simulink model "test"  (R2016b)
settings: Solver=ode3  StartTime=0.0  StopTime=inf  FixedStep=0.01  RelTol=1e-3  EnableMultiTasking=on
undefined symbols (not defined in the file): C, D, eps_c, k_cc, K_q1f, K_q1r, K_q2f, K_q2r, K_q3f, K_q3r, K_q4f, K_q4r, K_q5f, K_q5r, K_q6f, K_q6r, K_T1f, K_T1r, K_T2f, K_T2r, K_T3f, K_T3r, K_T4f, K_T4r, K_T5f, K_T5r, K_T6f, K_T6r, Max_rotation, Max_thrust, Min_thrust, n_c, p_cc, pwm_thr1_backward, pwm_thr1_forward, pwm_thr2_backward, pwm_thr2_forward, pwm_thr3_backward, pwm_thr3_forward, pwm_thr4_backward, pwm_thr4_forward, pwm_thr5_backward, pwm_thr5_forward, pwm_thr6_backward, pwm_thr6_forward, r_cc, Rho, Thruster
libraries: dspmtrx3 x9, marine_gnc x8, simulink_extras x3, simulink x1
(part 3 of 4)

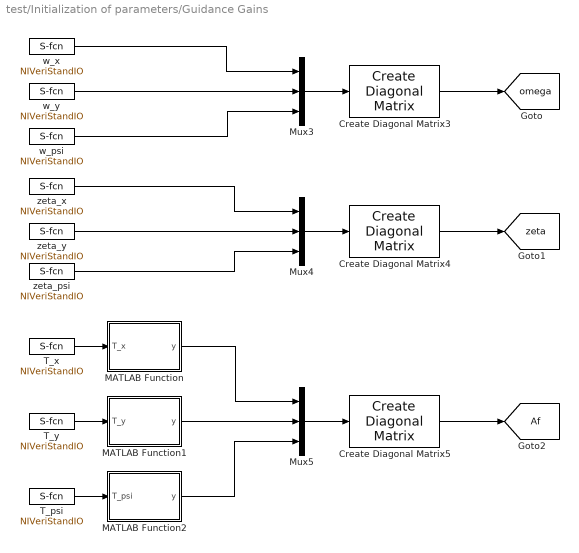
== system test/Initialization of parameters/Guidance Gains ==
  Create Diagonal Matrix3 : dspmtrx3/Create Diagonal Matrix
  Create Diagonal Matrix4 : dspmtrx3/Create Diagonal Matrix
  Create Diagonal Matrix5 : dspmtrx3/Create Diagonal Matrix
  MATLAB Function : MATLAB Function  TreatAsAtomicUnit=on
  MATLAB Function1 : MATLAB Function  TreatAsAtomicUnit=on
  MATLAB Function2 : MATLAB Function  TreatAsAtomicUnit=on
  Mux3 : Mux  Inputs=3
  Mux4 : Mux  Inputs=3
  Mux5 : Mux  Inputs=3
  T_psi : S-Function  Priority=7  FunctionName=NIVeriStandIO  Parameters=width dtype portnum stime stype btype  SFunctionDeploymentMode=off  EnableBusSupport=off  mask(NI VeriStand Inport){portnum=7, width=-1, stime=-1, dtype=auto, stype=auto, btype=1}
      mask prompts: portnum "Port number:"; width "Port dimensions (-1 for dynamically sized):"; stime "Sample time (-1 for inherited):"; dtype "Data type:"; stype "Signal type:"; btype "Block type:"
      mask help: Use this inport on any level of nested subsystems to allow NI VeriStand software to map signals to it.
      mask init:
      | NIVeriStandIO_init;
      settings: CopyFcn=NIVeriStand_MDL_functions('', 'IO_copy');  DeleteFcn=NIVeriStand_MDL_functions('', 'IO_delete');  MoveFcn=set_param(gcb, 'Mask', 'on');
      mask Callback portnum: NIVeriStand_MDL_functions('', 'IO_setportnum');
      mask TypeOptions dtype: auto | double | single | int8 | uint8 | int16 | uint16 | int32 | uint32 | boolean
      mask Callback dtype: NIVeriStand_MDL_functions('', 'IO_booleansignal');
      mask TypeOptions stype: auto | real | complex
      mask Display:
      | patch([-x x], [-y y], [.90980 .81960 .32156]);
      | plot([xrad -x x xrad], [yrad -y y yrad]);
      | fprintf('NI In%d', portnum);
  T_x : S-Function  Priority=8  FunctionName=NIVeriStandIO  Parameters=width dtype portnum stime stype btype  SFunctionDeploymentMode=off  EnableBusSupport=off  mask(NI VeriStand Inport){portnum=8, width=-1, stime=-1, dtype=auto, stype=auto, btype=1}
      mask prompts: portnum "Port number:"; width "Port dimensions (-1 for dynamically sized):"; stime "Sample time (-1 for inherited):"; dtype "Data type:"; stype "Signal type:"; btype "Block type:"
      mask help: Use this inport on any level of nested subsystems to allow NI VeriStand software to map signals to it.
      mask init:
      | NIVeriStandIO_init;
      settings: CopyFcn=NIVeriStand_MDL_functions('', 'IO_copy');  DeleteFcn=NIVeriStand_MDL_functions('', 'IO_delete');  MoveFcn=set_param(gcb, 'Mask', 'on');
      mask Callback portnum: NIVeriStand_MDL_functions('', 'IO_setportnum');
      mask TypeOptions dtype: auto | double | single | int8 | uint8 | int16 | uint16 | int32 | uint32 | boolean
      mask Callback dtype: NIVeriStand_MDL_functions('', 'IO_booleansignal');
      mask TypeOptions stype: auto | real | complex
      mask Display:
      | patch([-x x], [-y y], [.90980 .81960 .32156]);
      | plot([xrad -x x xrad], [yrad -y y yrad]);
      | fprintf('NI In%d', portnum);
  T_y : S-Function  Priority=9  FunctionName=NIVeriStandIO  Parameters=width dtype portnum stime stype btype  SFunctionDeploymentMode=off  EnableBusSupport=off  mask(NI VeriStand Inport){portnum=9, width=-1, stime=-1, dtype=auto, stype=auto, btype=1}
      mask prompts: portnum "Port number:"; width "Port dimensions (-1 for dynamically sized):"; stime "Sample time (-1 for inherited):"; dtype "Data type:"; stype "Signal type:"; btype "Block type:"
      mask help: Use this inport on any level of nested subsystems to allow NI VeriStand software to map signals to it.
      mask init:
      | NIVeriStandIO_init;
      settings: CopyFcn=NIVeriStand_MDL_functions('', 'IO_copy');  DeleteFcn=NIVeriStand_MDL_functions('', 'IO_delete');  MoveFcn=set_param(gcb, 'Mask', 'on');
      mask Callback portnum: NIVeriStand_MDL_functions('', 'IO_setportnum');
      mask TypeOptions dtype: auto | double | single | int8 | uint8 | int16 | uint16 | int32 | uint32 | boolean
      mask Callback dtype: NIVeriStand_MDL_functions('', 'IO_booleansignal');
      mask TypeOptions stype: auto | real | complex
      mask Display:
      | patch([-x x], [-y y], [.90980 .81960 .32156]);
      | plot([xrad -x x xrad], [yrad -y y yrad]);
      | fprintf('NI In%d', portnum);
  w_psi : S-Function  Priority=3  FunctionName=NIVeriStandIO  Parameters=width dtype portnum stime stype btype  SFunctionDeploymentMode=off  EnableBusSupport=off  mask(NI VeriStand Inport){portnum=3, width=-1, stime=-1, dtype=auto, stype=auto, btype=1}
      mask prompts: portnum "Port number:"; width "Port dimensions (-1 for dynamically sized):"; stime "Sample time (-1 for inherited):"; dtype "Data type:"; stype "Signal type:"; btype "Block type:"
      mask help: Use this inport on any level of nested subsystems to allow NI VeriStand software to map signals to it.
      mask init:
      | NIVeriStandIO_init;
      settings: CopyFcn=NIVeriStand_MDL_functions('', 'IO_copy');  DeleteFcn=NIVeriStand_MDL_functions('', 'IO_delete');  MoveFcn=set_param(gcb, 'Mask', 'on');
      mask Callback portnum: NIVeriStand_MDL_functions('', 'IO_setportnum');
      mask TypeOptions dtype: auto | double | single | int8 | uint8 | int16 | uint16 | int32 | uint32 | boolean
      mask Callback dtype: NIVeriStand_MDL_functions('', 'IO_booleansignal');
      mask TypeOptions stype: auto | real | complex
      mask Display:
      | patch([-x x], [-y y], [.90980 .81960 .32156]);
      | plot([xrad -x x xrad], [yrad -y y yrad]);
      | fprintf('NI In%d', portnum);
  w_x : S-Function  Priority=1  FunctionName=NIVeriStandIO  Parameters=width dtype portnum stime stype btype  SFunctionDeploymentMode=off  EnableBusSupport=off  mask(NI VeriStand Inport){portnum=1, width=-1, stime=-1, dtype=auto, stype=auto, btype=1}
      mask prompts: portnum "Port number:"; width "Port dimensions (-1 for dynamically sized):"; stime "Sample time (-1 for inherited):"; dtype "Data type:"; stype "Signal type:"; btype "Block type:"
      mask help: Use this inport on any level of nested subsystems to allow NI VeriStand software to map signals to it.
      mask init:
      | NIVeriStandIO_init;
      settings: CopyFcn=NIVeriStand_MDL_functions('', 'IO_copy');  DeleteFcn=NIVeriStand_MDL_functions('', 'IO_delete');  MoveFcn=set_param(gcb, 'Mask', 'on');
      mask Callback portnum: NIVeriStand_MDL_functions('', 'IO_setportnum');
      mask TypeOptions dtype: auto | double | single | int8 | uint8 | int16 | uint16 | int32 | uint32 | boolean
      mask Callback dtype: NIVeriStand_MDL_functions('', 'IO_booleansignal');
      mask TypeOptions stype: auto | real | complex
      mask Display:
      | patch([-x x], [-y y], [.90980 .81960 .32156]);
      | plot([xrad -x x xrad], [yrad -y y yrad]);
      | fprintf('NI In%d', portnum);
  w_y : S-Function  Priority=2  FunctionName=NIVeriStandIO  Parameters=width dtype portnum stime stype btype  SFunctionDeploymentMode=off  EnableBusSupport=off  mask(NI VeriStand Inport){portnum=2, width=-1, stime=-1, dtype=auto, stype=auto, btype=1}
      mask prompts: portnum "Port number:"; width "Port dimensions (-1 for dynamically sized):"; stime "Sample time (-1 for inherited):"; dtype "Data type:"; stype "Signal type:"; btype "Block type:"
      mask help: Use this inport on any level of nested subsystems to allow NI VeriStand software to map signals to it.
      mask init:
      | NIVeriStandIO_init;
      settings: CopyFcn=NIVeriStand_MDL_functions('', 'IO_copy');  DeleteFcn=NIVeriStand_MDL_functions('', 'IO_delete');  MoveFcn=set_param(gcb, 'Mask', 'on');
      mask Callback portnum: NIVeriStand_MDL_functions('', 'IO_setportnum');
      mask TypeOptions dtype: auto | double | single | int8 | uint8 | int16 | uint16 | int32 | uint32 | boolean
      mask Callback dtype: NIVeriStand_MDL_functions('', 'IO_booleansignal');
      mask TypeOptions stype: auto | real | complex
      mask Display:
      | patch([-x x], [-y y], [.90980 .81960 .32156]);
      | plot([xrad -x x xrad], [yrad -y y yrad]);
      | fprintf('NI In%d', portnum);
  zeta_psi : S-Function  Priority=4  FunctionName=NIVeriStandIO  Parameters=width dtype portnum stime stype btype  SFunctionDeploymentMode=off  EnableBusSupport=off  mask(NI VeriStand Inport){portnum=4, width=-1, stime=-1, dtype=auto, stype=auto, btype=1}
      mask prompts: portnum "Port number:"; width "Port dimensions (-1 for dynamically sized):"; stime "Sample time (-1 for inherited):"; dtype "Data type:"; stype "Signal type:"; btype "Block type:"
      mask help: Use this inport on any level of nested subsystems to allow NI VeriStand software to map signals to it.
      mask init:
      | NIVeriStandIO_init;
      settings: CopyFcn=NIVeriStand_MDL_functions('', 'IO_copy');  DeleteFcn=NIVeriStand_MDL_functions('', 'IO_delete');  MoveFcn=set_param(gcb, 'Mask', 'on');
      mask Callback portnum: NIVeriStand_MDL_functions('', 'IO_setportnum');
      mask TypeOptions dtype: auto | double | single | int8 | uint8 | int16 | uint16 | int32 | uint32 | boolean
      mask Callback dtype: NIVeriStand_MDL_functions('', 'IO_booleansignal');
      mask TypeOptions stype: auto | real | complex
      mask Display:
      | patch([-x x], [-y y], [.90980 .81960 .32156]);
      | plot([xrad -x x xrad], [yrad -y y yrad]);
      | fprintf('NI In%d', portnum);
  zeta_x : S-Function  Priority=5  FunctionName=NIVeriStandIO  Parameters=width dtype portnum stime stype btype  SFunctionDeploymentMode=off  EnableBusSupport=off  mask(NI VeriStand Inport){portnum=5, width=-1, stime=-1, dtype=auto, stype=auto, btype=1}
      mask prompts: portnum "Port number:"; width "Port dimensions (-1 for dynamically sized):"; stime "Sample time (-1 for inherited):"; dtype "Data type:"; stype "Signal type:"; btype "Block type:"
      mask help: Use this inport on any level of nested subsystems to allow NI VeriStand software to map signals to it.
      mask init:
      | NIVeriStandIO_init;
      settings: CopyFcn=NIVeriStand_MDL_functions('', 'IO_copy');  DeleteFcn=NIVeriStand_MDL_functions('', 'IO_delete');  MoveFcn=set_param(gcb, 'Mask', 'on');
      mask Callback portnum: NIVeriStand_MDL_functions('', 'IO_setportnum');
      mask TypeOptions dtype: auto | double | single | int8 | uint8 | int16 | uint16 | int32 | uint32 | boolean
      mask Callback dtype: NIVeriStand_MDL_functions('', 'IO_booleansignal');
      mask TypeOptions stype: auto | real | complex
      mask Display:
      | patch([-x x], [-y y], [.90980 .81960 .32156]);
      | plot([xrad -x x xrad], [yrad -y y yrad]);
      | fprintf('NI In%d', portnum);
  zeta_y : S-Function  Priority=6  FunctionName=NIVeriStandIO  Parameters=width dtype portnum stime stype btype  SFunctionDeploymentMode=off  EnableBusSupport=off  mask(NI VeriStand Inport){portnum=6, width=-1, stime=-1, dtype=auto, stype=auto, btype=1}
      mask prompts: portnum "Port number:"; width "Port dimensions (-1 for dynamically sized):"; stime "Sample time (-1 for inherited):"; dtype "Data type:"; stype "Signal type:"; btype "Block type:"
      mask help: Use this inport on any level of nested subsystems to allow NI VeriStand software to map signals to it.
      mask init:
      | NIVeriStandIO_init;
      settings: CopyFcn=NIVeriStand_MDL_functions('', 'IO_copy');  DeleteFcn=NIVeriStand_MDL_functions('', 'IO_delete');  MoveFcn=set_param(gcb, 'Mask', 'on');
      mask Callback portnum: NIVeriStand_MDL_functions('', 'IO_setportnum');
      mask TypeOptions dtype: auto | double | single | int8 | uint8 | int16 | uint16 | int32 | uint32 | boolean
      mask Callback dtype: NIVeriStand_MDL_functions('', 'IO_booleansignal');
      mask TypeOptions stype: auto | real | complex
      mask Display:
      | patch([-x x], [-y y], [.90980 .81960 .32156]);
      | plot([xrad -x x xrad], [yrad -y y yrad]);
      | fprintf('NI In%d', portnum);
  tag scope: Af=global, omega=global, zeta=global
  wires:
  w_x/1 -> Mux3/1
  w_psi/1 -> Mux3/3
  w_y/1 -> Mux3/2
  Mux3/1 -> Create Diagonal Matrix3/1
  Create Diagonal Matrix3/1 -> [omega]
  Mux4/1 -> Create Diagonal Matrix4/1
  T_x/1 -> MATLAB Function/1(T_x)
  T_psi/1 -> MATLAB Function2/1(T_psi)
  T_y/1 -> MATLAB Function1/1(T_y)
  Mux5/1 -> Create Diagonal Matrix5/1
  Create Diagonal Matrix4/1 -> [zeta]
  Create Diagonal Matrix5/1 -> [Af]
  zeta_x/1 -> Mux4/1
  zeta_y/1 -> Mux4/2
  zeta_psi/1 -> Mux4/3
  MATLAB Function/1(y) -> Mux5/1
  MATLAB Function1/1(y) -> Mux5/2
  MATLAB Function2/1(y) -> Mux5/3

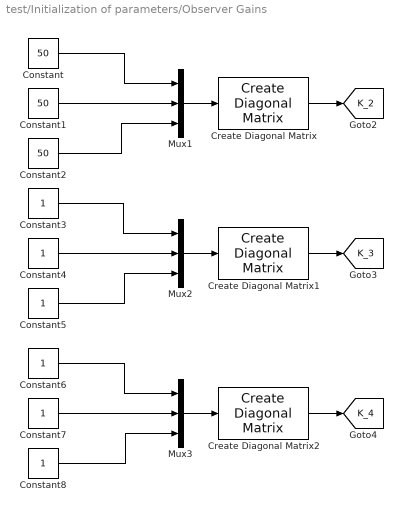
== system test/Initialization of parameters/Observer Gains ==
  Constant : Constant  Value=50
  Constant1 : Constant  Value=50
  Constant2 : Constant  Value=50
  Constant{3..8} (6 alike) : Constant
  Create Diagonal Matrix : dspmtrx3/Create Diagonal Matrix
  Create Diagonal Matrix1 : dspmtrx3/Create Diagonal Matrix
  Create Diagonal Matrix2 : dspmtrx3/Create Diagonal Matrix
  Mux1 : Mux  Inputs=3
  Mux2 : Mux  Inputs=3
  Mux3 : Mux  Inputs=3
  tag scope: K_2=global, K_3=global, K_4=global
  wires:
  Constant/1 -> Mux1/1
  Constant2/1 -> Mux1/3
  Constant1/1 -> Mux1/2
  Mux1/1 -> Create Diagonal Matrix/1
  Create Diagonal Matrix/1 -> [K_2]
  Constant3/1 -> Mux2/1
  Constant5/1 -> Mux2/3
  Constant4/1 -> Mux2/2
  Mux2/1 -> Create Diagonal Matrix1/1
  Constant8/1 -> Mux3/3
  Constant7/1 -> Mux3/2
  Mux3/1 -> Create Diagonal Matrix2/1
  Create Diagonal Matrix1/1 -> [K_3]
  Create Diagonal Matrix2/1 -> [K_4]
  Constant6/1 -> Mux3/1

== system test/Nonlinear Passisve Observer/Transpose Rotation Matrix ==
  psi : Inport
  y_tilde : Inport  Port=2
  Mux : Mux  Inputs=2
  Mux1 : Mux  Inputs=3
  Row1 : Fcn  Expr=cos(u(1))*u(2)+sin(u(1))*u(3)
  Row2 : Fcn  Expr=-sin(u(1))*u(2)+cos(u(1))*u(3)
  Row3 : Fcn  Expr=u(4)
  R(psi)'*y_tilde : Outport
  wires:
  Mux/1 -> Row3/1, Row2/1, Row1/1
  Row1/1 -> Mux1/1
  Row2/1 -> Mux1/2
  Row3/1 -> Mux1/3
  Mux1/1 -> R(psi)'*y_tilde/1
  psi/1 -> Mux/1
  y_tilde/1 -> Mux/2

== system test/Nonlinear Passisve Observer/Transpose Rotation matrix ==
  psi : Inport
  b_hat : Inport  Port=2
  Mux : Mux  Inputs=2
  Mux1 : Mux  Inputs=3
  Row1 : Fcn  Expr=cos(u(1))*u(2)+sin(u(1))*u(3)
  Row2 : Fcn  Expr=-sin(u(1))*u(2)+cos(u(1))*u(3)
  Row3 : Fcn  Expr=u(4)
  R(psi)'*b_hat : Outport
  wires:
  Mux/1 -> Row3/1, Row2/1, Row1/1
  Row1/1 -> Mux1/1
  Row2/1 -> Mux1/2
  Row3/1 -> Mux1/3
  Mux1/1 -> R(psi)'*b_hat/1
  psi/1 -> Mux/1
  b_hat/1 -> Mux/2

== system test/Observer output /b_hat output ==
  b_hat : Inport
  Demux : Demux  Outputs=3
  b_psi_hat : S-Function  Priority=3  FunctionName=NIVeriStandIO  Parameters=width dtype portnum stime stype btype  SFunctionDeploymentMode=off  EnableBusSupport=off  mask(NI VeriStand Outport){portnum=3, width=-1, stime=-1, dtype=auto, stype=auto, btype=0}
      mask prompts: portnum "Port number:"; width "Port dimensions (-1 for dynamically sized):"; stime "Sample time (-1 for inherited):"; dtype "Data type:"; stype "Signal type:"; btype "Block type:"
      mask help: Use this outport on any level of nested subsystems to allow NI VeriStand software to map signals to it.
      mask init:
      | NIVeriStandIO_init;
      settings: CopyFcn=NIVeriStand_MDL_functions('', 'IO_copy');  DeleteFcn=NIVeriStand_MDL_functions('', 'IO_delete');  MoveFcn=set_param(gcb, 'Mask', 'on');
      mask Callback portnum: NIVeriStand_MDL_functions('', 'IO_setportnum');
      mask TypeOptions dtype: auto | double | single | int8 | uint8 | int16 | uint16 | int32 | uint32 | boolean
      mask Callback dtype: NIVeriStand_MDL_functions('', 'IO_booleansignal');
      mask TypeOptions stype: auto | real | complex
      mask Display:
      | patch([-x x], [-y y], [.90980 .81960 .32156]);
      | plot([xrad -x x xrad], [yrad -y y yrad]);
      | fprintf('NI Out%d', portnum);
  b_x_hat : S-Function  Priority=1  FunctionName=NIVeriStandIO  Parameters=width dtype portnum stime stype btype  SFunctionDeploymentMode=off  EnableBusSupport=off  mask(NI VeriStand Outport){portnum=1, width=-1, stime=-1, dtype=auto, stype=auto, btype=0}
      mask prompts: portnum "Port number:"; width "Port dimensions (-1 for dynamically sized):"; stime "Sample time (-1 for inherited):"; dtype "Data type:"; stype "Signal type:"; btype "Block type:"
      mask help: Use this outport on any level of nested subsystems to allow NI VeriStand software to map signals to it.
      mask init:
      | NIVeriStandIO_init;
      settings: CopyFcn=NIVeriStand_MDL_functions('', 'IO_copy');  DeleteFcn=NIVeriStand_MDL_functions('', 'IO_delete');  MoveFcn=set_param(gcb, 'Mask', 'on');
      mask Callback portnum: NIVeriStand_MDL_functions('', 'IO_setportnum');
      mask TypeOptions dtype: auto | double | single | int8 | uint8 | int16 | uint16 | int32 | uint32 | boolean
      mask Callback dtype: NIVeriStand_MDL_functions('', 'IO_booleansignal');
      mask TypeOptions stype: auto | real | complex
      mask Display:
      | patch([-x x], [-y y], [.90980 .81960 .32156]);
      | plot([xrad -x x xrad], [yrad -y y yrad]);
      | fprintf('NI Out%d', portnum);
  b_y_hat : S-Function  Priority=2  FunctionName=NIVeriStandIO  Parameters=width dtype portnum stime stype btype  SFunctionDeploymentMode=off  EnableBusSupport=off  mask(NI VeriStand Outport){portnum=2, width=-1, stime=-1, dtype=auto, stype=auto, btype=0}
      mask prompts: portnum "Port number:"; width "Port dimensions (-1 for dynamically sized):"; stime "Sample time (-1 for inherited):"; dtype "Data type:"; stype "Signal type:"; btype "Block type:"
      mask help: Use this outport on any level of nested subsystems to allow NI VeriStand software to map signals to it.
      mask init:
      | NIVeriStandIO_init;
      settings: CopyFcn=NIVeriStand_MDL_functions('', 'IO_copy');  DeleteFcn=NIVeriStand_MDL_functions('', 'IO_delete');  MoveFcn=set_param(gcb, 'Mask', 'on');
      mask Callback portnum: NIVeriStand_MDL_functions('', 'IO_setportnum');
      mask TypeOptions dtype: auto | double | single | int8 | uint8 | int16 | uint16 | int32 | uint32 | boolean
      mask Callback dtype: NIVeriStand_MDL_functions('', 'IO_booleansignal');
      mask TypeOptions stype: auto | real | complex
      mask Display:
      | patch([-x x], [-y y], [.90980 .81960 .32156]);
      | plot([xrad -x x xrad], [yrad -y y yrad]);
      | fprintf('NI Out%d', portnum);
  wires:
  Demux/1 -> b_x_hat/1
  Demux/2 -> b_y_hat/1
  Demux/3 -> b_psi_hat/1
  b_hat/1 -> Demux/1

== system test/Observer output /eta_hat output ==
  eta-_hat : Inport
  Demux : Demux  Outputs=3
  psi_hat : S-Function  Priority=3  FunctionName=NIVeriStandIO  Parameters=width dtype portnum stime stype btype  SFunctionDeploymentMode=off  EnableBusSupport=off  mask(NI VeriStand Outport){portnum=3, width=-1, stime=-1, dtype=auto, stype=auto, btype=0}
      mask prompts: portnum "Port number:"; width "Port dimensions (-1 for dynamically sized):"; stime "Sample time (-1 for inherited):"; dtype "Data type:"; stype "Signal type:"; btype "Block type:"
      mask help: Use this outport on any level of nested subsystems to allow NI VeriStand software to map signals to it.
      mask init:
      | NIVeriStandIO_init;
      settings: CopyFcn=NIVeriStand_MDL_functions('', 'IO_copy');  DeleteFcn=NIVeriStand_MDL_functions('', 'IO_delete');  MoveFcn=set_param(gcb, 'Mask', 'on');
      mask Callback portnum: NIVeriStand_MDL_functions('', 'IO_setportnum');
      mask TypeOptions dtype: auto | double | single | int8 | uint8 | int16 | uint16 | int32 | uint32 | boolean
      mask Callback dtype: NIVeriStand_MDL_functions('', 'IO_booleansignal');
      mask TypeOptions stype: auto | real | complex
      mask Display:
      | patch([-x x], [-y y], [.90980 .81960 .32156]);
      | plot([xrad -x x xrad], [yrad -y y yrad]);
      | fprintf('NI Out%d', portnum);
  x_hat : S-Function  Priority=1  FunctionName=NIVeriStandIO  Parameters=width dtype portnum stime stype btype  SFunctionDeploymentMode=off  EnableBusSupport=off  mask(NI VeriStand Outport){portnum=1, width=-1, stime=-1, dtype=auto, stype=auto, btype=0}
      mask prompts: portnum "Port number:"; width "Port dimensions (-1 for dynamically sized):"; stime "Sample time (-1 for inherited):"; dtype "Data type:"; stype "Signal type:"; btype "Block type:"
      mask help: Use this outport on any level of nested subsystems to allow NI VeriStand software to map signals to it.
      mask init:
      | NIVeriStandIO_init;
      settings: CopyFcn=NIVeriStand_MDL_functions('', 'IO_copy');  DeleteFcn=NIVeriStand_MDL_functions('', 'IO_delete');  MoveFcn=set_param(gcb, 'Mask', 'on');
      mask Callback portnum: NIVeriStand_MDL_functions('', 'IO_setportnum');
      mask TypeOptions dtype: auto | double | single | int8 | uint8 | int16 | uint16 | int32 | uint32 | boolean
      mask Callback dtype: NIVeriStand_MDL_functions('', 'IO_booleansignal');
      mask TypeOptions stype: auto | real | complex
      mask Display:
      | patch([-x x], [-y y], [.90980 .81960 .32156]);
      | plot([xrad -x x xrad], [yrad -y y yrad]);
      | fprintf('NI Out%d', portnum);
  y_hat : S-Function  Priority=2  FunctionName=NIVeriStandIO  Parameters=width dtype portnum stime stype btype  SFunctionDeploymentMode=off  EnableBusSupport=off  mask(NI VeriStand Outport){portnum=2, width=-1, stime=-1, dtype=auto, stype=auto, btype=0}
      mask prompts: portnum "Port number:"; width "Port dimensions (-1 for dynamically sized):"; stime "Sample time (-1 for inherited):"; dtype "Data type:"; stype "Signal type:"; btype "Block type:"
      mask help: Use this outport on any level of nested subsystems to allow NI VeriStand software to map signals to it.
      mask init:
      | NIVeriStandIO_init;
      settings: CopyFcn=NIVeriStand_MDL_functions('', 'IO_copy');  DeleteFcn=NIVeriStand_MDL_functions('', 'IO_delete');  MoveFcn=set_param(gcb, 'Mask', 'on');
      mask Callback portnum: NIVeriStand_MDL_functions('', 'IO_setportnum');
      mask TypeOptions dtype: auto | double | single | int8 | uint8 | int16 | uint16 | int32 | uint32 | boolean
      mask Callback dtype: NIVeriStand_MDL_functions('', 'IO_booleansignal');
      mask TypeOptions stype: auto | real | complex
      mask Display:
      | patch([-x x], [-y y], [.90980 .81960 .32156]);
      | plot([xrad -x x xrad], [yrad -y y yrad]);
      | fprintf('NI Out%d', portnum);
  wires:
  Demux/1 -> x_hat/1
  Demux/2 -> y_hat/1
  Demux/3 -> psi_hat/1
  eta-_hat/1 -> Demux/1

== system test/Observer output /nu_dot_hat output ==
  nu_dot_hat : Inport
  Demux : Demux  Outputs=3
  r_dot_hat : S-Function  Priority=3  FunctionName=NIVeriStandIO  Parameters=width dtype portnum stime stype btype  SFunctionDeploymentMode=off  EnableBusSupport=off  mask(NI VeriStand Outport){portnum=3, width=-1, stime=-1, dtype=auto, stype=auto, btype=0}
      mask prompts: portnum "Port number:"; width "Port dimensions (-1 for dynamically sized):"; stime "Sample time (-1 for inherited):"; dtype "Data type:"; stype "Signal type:"; btype "Block type:"
      mask help: Use this outport on any level of nested subsystems to allow NI VeriStand software to map signals to it.
      mask init:
      | NIVeriStandIO_init;
      settings: CopyFcn=NIVeriStand_MDL_functions('', 'IO_copy');  DeleteFcn=NIVeriStand_MDL_functions('', 'IO_delete');  MoveFcn=set_param(gcb, 'Mask', 'on');
      mask Callback portnum: NIVeriStand_MDL_functions('', 'IO_setportnum');
      mask TypeOptions dtype: auto | double | single | int8 | uint8 | int16 | uint16 | int32 | uint32 | boolean
      mask Callback dtype: NIVeriStand_MDL_functions('', 'IO_booleansignal');
      mask TypeOptions stype: auto | real | complex
      mask Display:
      | patch([-x x], [-y y], [.90980 .81960 .32156]);
      | plot([xrad -x x xrad], [yrad -y y yrad]);
      | fprintf('NI Out%d', portnum);
  u_dot_hat : S-Function  Priority=1  FunctionName=NIVeriStandIO  Parameters=width dtype portnum stime stype btype  SFunctionDeploymentMode=off  EnableBusSupport=off  mask(NI VeriStand Outport){portnum=1, width=-1, stime=-1, dtype=auto, stype=auto, btype=0}
      mask prompts: portnum "Port number:"; width "Port dimensions (-1 for dynamically sized):"; stime "Sample time (-1 for inherited):"; dtype "Data type:"; stype "Signal type:"; btype "Block type:"
      mask help: Use this outport on any level of nested subsystems to allow NI VeriStand software to map signals to it.
      mask init:
      | NIVeriStandIO_init;
      settings: CopyFcn=NIVeriStand_MDL_functions('', 'IO_copy');  DeleteFcn=NIVeriStand_MDL_functions('', 'IO_delete');  MoveFcn=set_param(gcb, 'Mask', 'on');
      mask Callback portnum: NIVeriStand_MDL_functions('', 'IO_setportnum');
      mask TypeOptions dtype: auto | double | single | int8 | uint8 | int16 | uint16 | int32 | uint32 | boolean
      mask Callback dtype: NIVeriStand_MDL_functions('', 'IO_booleansignal');
      mask TypeOptions stype: auto | real | complex
      mask Display:
      | patch([-x x], [-y y], [.90980 .81960 .32156]);
      | plot([xrad -x x xrad], [yrad -y y yrad]);
      | fprintf('NI Out%d', portnum);
  v_dot_hat : S-Function  Priority=2  FunctionName=NIVeriStandIO  Parameters=width dtype portnum stime stype btype  SFunctionDeploymentMode=off  EnableBusSupport=off  mask(NI VeriStand Outport){portnum=2, width=-1, stime=-1, dtype=auto, stype=auto, btype=0}
      mask prompts: portnum "Port number:"; width "Port dimensions (-1 for dynamically sized):"; stime "Sample time (-1 for inherited):"; dtype "Data type:"; stype "Signal type:"; btype "Block type:"
      mask help: Use this outport on any level of nested subsystems to allow NI VeriStand software to map signals to it.
      mask init:
      | NIVeriStandIO_init;
      settings: CopyFcn=NIVeriStand_MDL_functions('', 'IO_copy');  DeleteFcn=NIVeriStand_MDL_functions('', 'IO_delete');  MoveFcn=set_param(gcb, 'Mask', 'on');
      mask Callback portnum: NIVeriStand_MDL_functions('', 'IO_setportnum');
      mask TypeOptions dtype: auto | double | single | int8 | uint8 | int16 | uint16 | int32 | uint32 | boolean
      mask Callback dtype: NIVeriStand_MDL_functions('', 'IO_booleansignal');
      mask TypeOptions stype: auto | real | complex
      mask Display:
      | patch([-x x], [-y y], [.90980 .81960 .32156]);
      | plot([xrad -x x xrad], [yrad -y y yrad]);
      | fprintf('NI Out%d', portnum);
  wires:
  Demux/1 -> u_dot_hat/1
  Demux/2 -> v_dot_hat/1
  Demux/3 -> r_dot_hat/1
  nu_dot_hat/1 -> Demux/1

== system test/Observer output /nu_hat output ==
  nu_hat : Inport
  Demux : Demux  Outputs=3
  r_hat : S-Function  Priority=3  FunctionName=NIVeriStandIO  Parameters=width dtype portnum stime stype btype  SFunctionDeploymentMode=off  EnableBusSupport=off  mask(NI VeriStand Outport){portnum=3, width=-1, stime=-1, dtype=auto, stype=auto, btype=0}
      mask prompts: portnum "Port number:"; width "Port dimensions (-1 for dynamically sized):"; stime "Sample time (-1 for inherited):"; dtype "Data type:"; stype "Signal type:"; btype "Block type:"
      mask help: Use this outport on any level of nested subsystems to allow NI VeriStand software to map signals to it.
      mask init:
      | NIVeriStandIO_init;
      settings: CopyFcn=NIVeriStand_MDL_functions('', 'IO_copy');  DeleteFcn=NIVeriStand_MDL_functions('', 'IO_delete');  MoveFcn=set_param(gcb, 'Mask', 'on');
      mask Callback portnum: NIVeriStand_MDL_functions('', 'IO_setportnum');
      mask TypeOptions dtype: auto | double | single | int8 | uint8 | int16 | uint16 | int32 | uint32 | boolean
      mask Callback dtype: NIVeriStand_MDL_functions('', 'IO_booleansignal');
      mask TypeOptions stype: auto | real | complex
      mask Display:
      | patch([-x x], [-y y], [.90980 .81960 .32156]);
      | plot([xrad -x x xrad], [yrad -y y yrad]);
      | fprintf('NI Out%d', portnum);
  u_hat : S-Function  Priority=1  FunctionName=NIVeriStandIO  Parameters=width dtype portnum stime stype btype  SFunctionDeploymentMode=off  EnableBusSupport=off  mask(NI VeriStand Outport){portnum=1, width=-1, stime=-1, dtype=auto, stype=auto, btype=0}
      mask prompts: portnum "Port number:"; width "Port dimensions (-1 for dynamically sized):"; stime "Sample time (-1 for inherited):"; dtype "Data type:"; stype "Signal type:"; btype "Block type:"
      mask help: Use this outport on any level of nested subsystems to allow NI VeriStand software to map signals to it.
      mask init:
      | NIVeriStandIO_init;
      settings: CopyFcn=NIVeriStand_MDL_functions('', 'IO_copy');  DeleteFcn=NIVeriStand_MDL_functions('', 'IO_delete');  MoveFcn=set_param(gcb, 'Mask', 'on');
      mask Callback portnum: NIVeriStand_MDL_functions('', 'IO_setportnum');
      mask TypeOptions dtype: auto | double | single | int8 | uint8 | int16 | uint16 | int32 | uint32 | boolean
      mask Callback dtype: NIVeriStand_MDL_functions('', 'IO_booleansignal');
      mask TypeOptions stype: auto | real | complex
      mask Display:
      | patch([-x x], [-y y], [.90980 .81960 .32156]);
      | plot([xrad -x x xrad], [yrad -y y yrad]);
      | fprintf('NI Out%d', portnum);
  v_hat : S-Function  Priority=2  FunctionName=NIVeriStandIO  Parameters=width dtype portnum stime stype btype  SFunctionDeploymentMode=off  EnableBusSupport=off  mask(NI VeriStand Outport){portnum=2, width=-1, stime=-1, dtype=auto, stype=auto, btype=0}
      mask prompts: portnum "Port number:"; width "Port dimensions (-1 for dynamically sized):"; stime "Sample time (-1 for inherited):"; dtype "Data type:"; stype "Signal type:"; btype "Block type:"
      mask help: Use this outport on any level of nested subsystems to allow NI VeriStand software to map signals to it.
      mask init:
      | NIVeriStandIO_init;
      settings: CopyFcn=NIVeriStand_MDL_functions('', 'IO_copy');  DeleteFcn=NIVeriStand_MDL_functions('', 'IO_delete');  MoveFcn=set_param(gcb, 'Mask', 'on');
      mask Callback portnum: NIVeriStand_MDL_functions('', 'IO_setportnum');
      mask TypeOptions dtype: auto | double | single | int8 | uint8 | int16 | uint16 | int32 | uint32 | boolean
      mask Callback dtype: NIVeriStand_MDL_functions('', 'IO_booleansignal');
      mask TypeOptions stype: auto | real | complex
      mask Display:
      | patch([-x x], [-y y], [.90980 .81960 .32156]);
      | plot([xrad -x x xrad], [yrad -y y yrad]);
      | fprintf('NI Out%d', portnum);
  wires:
  Demux/1 -> u_hat/1
  Demux/2 -> v_hat/1
  Demux/3 -> r_hat/1
  nu_hat/1 -> Demux/1

== system test/Thrust allocation/Optimal angle path and constraints on rotation speed ==
  Desired Angle : Inport  Partition=on  PartitionDimension=1  PartitionWidth=1
  "initial angle " : Inport  Port=2  Partition=on  PartitionDimension=1  PartitionWidth=1
  reset : Inport  Port=3  Partition=on  PartitionDimension=1  PartitionWidth=1
  Degrees to Radians : simulink_extras/Transformations/Degrees to Radians
  Delay : Delay  DelayLength=1  InitialCondition=0
  Ensuring angle is [-pi pi] : MATLAB Function  TreatAsAtomicUnit=on
  For Each : ForEach  DisableCoverage=on  IndexMode=One-based
  Integrator : Integrator  ExternalReset=either  InitialConditionSource=external
  MATLAB Function1 : MATLAB Function  TreatAsAtomicUnit=on
  Max Rotation Rate : Saturate  UpperLimit=Max_rotation  LowerLimit=-Max_rotation
  commanded Angle : Outport  ConcatenationDimension=1
  wires:
  Degrees to Radians/1 -> Ensuring angle is [-pi pi]/1(angle)
  Ensuring angle is [-pi pi]/1(y) -> commanded Angle/1
  Integrator/1 -> Delay/1, Degrees to Radians/1  "angle"
  "initial angle "/1 -> Integrator/3
  MATLAB Function1/1(psi_D) -> Max Rotation Rate/1
  Desired Angle/1 -> MATLAB Function1/1(desired)
  Delay/1 -> MATLAB Function1/2(actual)
  reset/1 -> Integrator/2
  Max Rotation Rate/1 -> Integrator/1

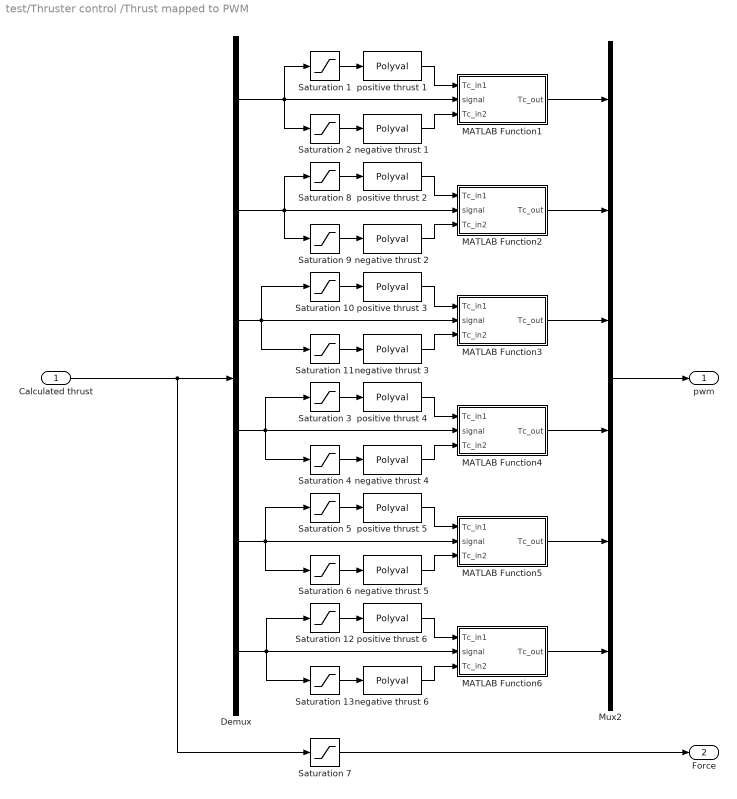
== system test/Thruster control /Thrust mapped to PWM ==
  Calculated thrust : Inport
  Demux : Demux  Outputs=6
  MATLAB Function1 : MATLAB Function  TreatAsAtomicUnit=on
  MATLAB Function2 : MATLAB Function  TreatAsAtomicUnit=on
  MATLAB Function3 : MATLAB Function  TreatAsAtomicUnit=on
  MATLAB Function4 : MATLAB Function  TreatAsAtomicUnit=on
  MATLAB Function5 : MATLAB Function  TreatAsAtomicUnit=on
  MATLAB Function6 : MATLAB Function  TreatAsAtomicUnit=on
  Mux2 : Mux  Inputs=6
  Saturation {1,3,5,8,10,12} (6 alike) : Saturate  UpperLimit=Max_thrust  LowerLimit=0
  Saturation {2,4,6,9,11,13} (6 alike) : Saturate  UpperLimit=0  LowerLimit=Min_thrust
  Saturation 7 : Saturate  UpperLimit=Max_thrust  LowerLimit=-Max_thrust
  negative thrust 1 : Polyval  Coefs=pwm_thr1_backward
  negative thrust 2 : Polyval  Coefs=pwm_thr2_backward
  negative thrust 3 : Polyval  Coefs=pwm_thr3_backward
  negative thrust 4 : Polyval  Coefs=pwm_thr4_backward
  negative thrust 5 : Polyval  Coefs=pwm_thr5_backward
  negative thrust 6 : Polyval  Coefs=pwm_thr6_backward
  positive thrust 1 : Polyval  Coefs=pwm_thr1_forward
  positive thrust 2 : Polyval  Coefs=pwm_thr2_forward
  positive thrust 3 : Polyval  Coefs=pwm_thr3_forward
  positive thrust 4 : Polyval  Coefs=pwm_thr4_forward
  positive thrust 5 : Polyval  Coefs=pwm_thr5_forward
  positive thrust 6 : Polyval  Coefs=pwm_thr6_forward
  pwm : Outport
  Force : Outport  Port=2
  wires:
  Mux2/1 -> pwm/1
  Calculated thrust/1 -> Saturation 7/1, Demux/1
  Saturation 7/1 -> Force/1
  positive thrust 1/1 -> MATLAB Function1/1(Tc_in1)
  negative thrust 1/1 -> MATLAB Function1/3(Tc_in2)
  Demux/1 -> Saturation 1/1, MATLAB Function1/2(signal), Saturation 2/1
  MATLAB Function1/1(Tc_out) -> Mux2/1
  Saturation 1/1 -> positive thrust 1/1
  Saturation 2/1 -> negative thrust 1/1
  positive thrust 2/1 -> MATLAB Function2/1(Tc_in1)
  negative thrust 2/1 -> MATLAB Function2/3(Tc_in2)
  Demux/2 -> Saturation 9/1, Saturation 8/1, MATLAB Function2/2(signal)
  MATLAB Function2/1(Tc_out) -> Mux2/2
  Saturation 8/1 -> positive thrust 2/1
  Saturation 9/1 -> negative thrust 2/1
  positive thrust 3/1 -> MATLAB Function3/1(Tc_in1)
  negative thrust 3/1 -> MATLAB Function3/3(Tc_in2)
  Demux/3 -> Saturation 11/1, MATLAB Function3/2(signal), Saturation 10/1
  MATLAB Function3/1(Tc_out) -> Mux2/3
  Saturation 10/1 -> positive thrust 3/1
  Saturation 11/1 -> negative thrust 3/1
  positive thrust 4/1 -> MATLAB Function4/1(Tc_in1)
  negative thrust 4/1 -> MATLAB Function4/3(Tc_in2)
  MATLAB Function4/1(Tc_out) -> Mux2/4
  Saturation 3/1 -> positive thrust 4/1
  Saturation 4/1 -> negative thrust 4/1
  Demux/4 -> Saturation 3/1, Saturation 4/1, MATLAB Function4/2(signal)
  positive thrust 5/1 -> MATLAB Function5/1(Tc_in1)
  negative thrust 5/1 -> MATLAB Function5/3(Tc_in2)
  MATLAB Function5/1(Tc_out) -> Mux2/5
  Saturation 5/1 -> positive thrust 5/1
  Saturation 6/1 -> negative thrust 5/1
  Demux/5 -> Saturation 5/1, MATLAB Function5/2(signal), Saturation 6/1
  positive thrust 6/1 -> MATLAB Function6/1(Tc_in1)
  negative thrust 6/1 -> MATLAB Function6/3(Tc_in2)
  MATLAB Function6/1(Tc_out) -> Mux2/6
  Saturation 12/1 -> positive thrust 6/1
  Saturation 13/1 -> negative thrust 6/1
  Demux/6 -> Saturation 13/1, Saturation 12/1, MATLAB Function6/2(signal)

== matlab function test/Referance/MATLAB Function ==
  data: omega input; y output; zeta input
function y = fcn(omega,zeta)

y = 2*zeta*omega;

== matlab function test/Referance/MATLAB Function1 ==
  data: omega input; y output; zeta input
function y = fcn(omega,zeta)

y = 2*zeta*omega;

== matlab function test/Referance/MATLAB Function2 ==
  data: omega input; y output
function y = fcn(omega)

y = omega*omega;

== matlab function test/Thrust allocation/Optimal angle path and constraints on rotation speed/Ensuring angle is [-pi pi] ==
  data: angle input; y output
function y = rad2pipi(angle)
% RAD2PIPI Converts an angle in rad to the interval (-pi pi]
%          Should be applied to all heading errors in a feedback control system
%          in order to avoid discontinuities.
%
% Author:     Roger Skjetne
% Date:       2003-09-05
% Revisions:  2004-09-02 Thor I. Fossen - replaced input argument x with angle
%             2005-01-05 Thor I. Fossen - ouput argument is set to y and not angle
%             2005-04-13 Roger Skjetne  - changed the function s in order
%                                         to account for correct mapping to
%                                         (-pi pi].
%
% ________________________________________________________________
%
% MSS GNC is a Matlab toolbox for guidance, navigation and control.
% The toolbox is part of the Marine Systems Simulator (MSS).
%
% Copyright (C) 2008 Thor I. Fossen and Tristan Perez
% 
% This program is free software: you can redistribute it and/or modify
% it under the terms of the GNU General Public License as published by
% the Free Software Foundation, either version 3 of the License, or
% (at your option) any later version.
% 
% This program is distributed in the hope that it will be useful, but
% WITHOUT ANY WARRANTY; without even the implied warranty of
% MERCHANTABILITY or FITNESS FOR A PARTICULAR PURPOSE.  See the 
% GNU General Public License for more details.
% 
% You should have received a copy of the GNU General Public License
% along with this program.  If not, see <http://www.gnu.org/licenses/>.
% 
% E-mail: contact@marinecontrol.org
% URL:    <http://www.marinecontrol.org>


% convert angle in rad to the interval <-pi pi> 
r = rem(angle+sign(angle)*pi,2*pi);
s = sign(sign(angle) + 2*(sign(abs(rem(angle+pi,2*pi)/(2*pi)))-1));
% s = sign(angle);

y = r - s*pi;

== matlab function test/Thruster control /Thrust mapped to PWM/MATLAB Function1 ==
  data: Tc_in1 input; signal input; Tc_out output; Tc_in2 input
function Tc_out = fcn(Tc_in1,signal,Tc_in2)
%#codegen

if signal >= 0
    Tc_out = Tc_in1;
else %signal < 0
    Tc_out = Tc_in2;
end

== matlab function test/Thrust allocation/Optimal angle path and constraints on rotation speed/MATLAB Function1 ==
  data: desired input; psi_D output; actual input
function psi_D   = fcn(desired,actual)
%#codegen
psi_D = desired-actual;
if abs(psi_D) >= 360
    psi_D = rem(psi_D,360);
end

if abs(psi_D) >= 180
    psi_D = psi_D - sign(psi_D)*360;
end

% if desired < 0 %&& abs(desired+actual) > 180
%     y = actual+360;
% else
%     y = abs(actual);
% end

%if desired-actual > 180
%    u = desired - 360;
%elseif desired-actual <= -180
%    u=actual + 360 ;
%else
%    u=desired;        
%end

end

%rotation = change-actual;% - actual; % If positive with clock, Negative against clock
%if rotation >= 180 || rotation <= -180
% u = desired;
%else 
%     u = actual;
%end

%change = abs(actual);

% if actual-desired > 180 && desired > 0 && rotation > 0
%     u = -180;
% elseif  actual-desired > 180 && desired > 0 && rotation < 0
%     u = 180;
% else 
%     u = actual;
% end

% if change > abs(desired-actual)
%     u = -actual;
% else
%     u = actual;
% end
% if desired >= 0.98*actual || desired <= -0.98*actual 
%     u = desired;
% else 
%     u = actual; 
% end
% paths = [abs(actual-desired),abs(-1*actual-desired)];
% fastest = min(paths);
% if paths(1) > paths(2)
%     fastest = paths(2);
% elseif paths(1) < paths(2)
%     fastest = paths(1);
% end
% % if desired > 0 && actual < 0 || desired < 0 && actual < 0
% % u = fastest;
% % elseif desired > 0 && actual > 0 || desired < 0 && actual < 0
% %     u = fastest;
% if desired-actual > 180 || desired-actual < -180
%     u = -actual;
% else 
%     u = actual;
% end

== matlab function test/Thrust allocation/MATLAB Function ==
  data: u input; sys output; ThrusterPosX input; ThrusterPosY input; C input
function sys = fcn(u,ThrusterPosX,ThrusterPosY,C)
% Complete system goes here!
Alpha1 = zeros(1,6);    % Allocating dimensions for faster computing
% Parameters thrusters
tc =  [u(1),u(2),u(3)]'; 
alpha = [u(4),u(5),u(6),u(7),u(8),u(9)]';

% Constraints for Thruster-Thruster interaction. Can be seen in "Initfile"
% how they are found
C1 = C(1,:);
C2 = C(2,:);
C3 = C(3,:);
C4 = C(4,:);
C5 = C(5,:);
C6 = C(6,:);

K = ones(1,6);

if alpha(1) < C1(1)-0.1  && alpha(1) > C1(2)+0.1 || alpha(1) > C1(3)+0.1 && alpha(1) < C1(4)-0.1
    K(1) = 0;
else 
    K(1) = K(1);
end

if alpha(2) > C2(1)-0.1  && alpha(2) < C2(2)+0.1 || alpha(2) > C2(3)-0.1 && alpha(2) < C2(4)+0.1
    K(2) = 0;
else 
    K(2) = K(2);
end

if alpha(3) < C3(1)+0.1  && alpha(3) > C3(2)-0.1 || alpha(3) < C3(3)+0.1 && alpha(3) > C3(4)-0.1
    K(3) = 0;
else 
    K(3) = K(3);
end

if alpha(4) > C4(1)+0.1  && alpha(4) < C4(2)-0.1 || alpha(4) < C4(3)-0.1 && alpha(4) > C4(4)+0.1
    K(4) = 0;
else 
    K(4) = K(4);
end

if alpha(5) < C5(1)-0.1  && alpha(5) > C5(2)+0.1 || alpha(5) < C5(3)-0.1 && alpha(5) > C5(4)+0.1
    K(5) = 0;
else 
    K(5) = K(5);
end

if alpha(6) > C6(1)+0.1  && alpha(6) < C6(2)-0.1 || alpha(6) > C6(3)+0.1 && alpha(6) < C6(4)-0.1
    K(6) = 0;
else 
    K(6) = K(6);
end

epsilon = u(10);

n_t = length(ThrusterPosX); % number of thrusters
B_surge = zeros(n_t,1); % Shells for faster computing
B_sway = zeros(n_t,1);  % Shells for faster computing
B_yaw = zeros(n_t,1);   % Shells for faster computing

for i = 1:1:n_t
  B_surge(i) = cosd(alpha(i));     %Thrust in x-direction for cartesian
  B_sway(i) = sind(alpha(i));      %Thrust in y-direction for cartesian
  B_yaw(i) = (sind(alpha(i))*ThrusterPosX(i) - cosd(alpha(i))*ThrusterPosY(i));
end


B = [B_surge,B_sway,B_yaw]';
B = B*diag(K); 
[U_singular,S_singular,V_singular] = svd(B,'econ');
S_singular_cross = 1./S_singular;
S_singular_cross(~isfinite(S_singular_cross))=0;
 if (S_singular_cross(3,3)>10*S_singular_cross(2,2)) 
     S_singular_cross(3,3)=0;
 end
 
u_optimized = V_singular*S_singular_cross*U_singular';

u_d = u_optimized*tc;          % Optimized Thrust



Te = [1 0 1 0 1 0 1 0 1 0 1 0;
      0 1 0 1 0 1 0 1 0 1 0 1;
      ThrusterPosY(1) ThrusterPosX(1) ThrusterPosY(2) ThrusterPosX(2) ThrusterPosY(3) ThrusterPosX(3) ...
      ThrusterPosY(4) ThrusterPosX(4) ThrusterPosY(5) ThrusterPosX(5) ThrusterPosY(6) ThrusterPosX(6)];

[U_singular2,S_singular2,V_singular2] = svd(Te,'econ');
S_singular_cross2 = 1./S_singular2;
S_singular_cross2(~isfinite(S_singular_cross2))=0;
 if (S_singular_cross2(3,3)>2*S_singular_cross2(2,2)) 
     S_singular_cross2(3,3)=0;
 end
T0 = V_singular2*S_singular_cross2*U_singular2'*tc;

alpha1 = [atan2d(T0(2),T0(1)) atan2d(T0(4),T0(3)) atan2d(T0(6),T0(5)) atan2d(T0(8),T0(7)) atan2d(T0(10),T0(9)) atan2d(T0(12),T0(11))];


%% Constraints
% Thruster 1 OK
%C1 = [151 130 -151 -130 ];
if alpha1(1) < C1(1)  && alpha1(1) > C1(2) && u_d(1) > 0 || alpha1(1) < C1(1)  && alpha1(1) > C1(2) && u_d(1) < 0
    c1 = [C1(1) C1(2)];
    [C_1,alpha_new1] = min(abs(c1-alpha1(1)));
    Alpha1(1) = c1(alpha_new1);
elseif alpha1(1) > C1(3) && alpha1(1) < C1(4) && u_d(1) > 0 || alpha1(1) > C1(3) && alpha1(1) < C1(4) && u_d(1) < 0
    c1 = [C1(3) C1(4)];
    [C_1,alpha_new1] = min(abs(c1-alpha1(1)));
    Alpha1(1) = c1(alpha_new1);
else 
    Alpha1(1) = alpha1(1);
end
if alpha(1) < C1(1)-0.1  && alpha(1) > C1(2)+0.1 || alpha(1) > C1(3)+0.1 && alpha(1) < C1(4)-0.1
    u_d(1) = 0;
else 
    u_d(1) = u_d(1);
end

% Thruster 2 
%C2 = [-99.85 -80.15 -50 -29];
if alpha1(2) < C2(1)  && alpha1(2) > C2(2) && u_d(2) > 0 || alpha1(2) < C2(1)  && alpha1(2) > C2(2) && u_d(2) < 0 
    c2 = [C2(1) C2(2)];
    [C_2,alpha_new2] = min(abs(c2-alpha1(2)));
    Alpha1(2) = c2(alpha_new2);
elseif alpha1(2) < C2(3) && alpha1(2) > C2(4) && u_d(2) > 0 || alpha1(2) < C2(3) && alpha1(2) > C2(4) && u_d(2) < 0
    c2 = [C2(3) C2(4)];
    [C_2,alpha_new2] = min(abs(c2-alpha1(2)));
    Alpha1(2) = c2(alpha_new2);
else 
    Alpha1(2) = alpha1(2);
end
if alpha(2) < C2(1)-0.1  && alpha(2) > C2(2)+0.1 || alpha(2) < C2(3)-0.1 && alpha(2) > C2(4)+0.1
    u_d(2) = 0;
else 
    u_d(2) = u_d(2);
end

% Thruster 3 
% C3 = [99.85 80.15 50 29]; 

if alpha1(3) > C3(1)  && alpha1(3) < C3(2) && u_d(3) > 0 || alpha1(3) > C3(1)  && alpha1(3) < C3(2) && u_d(3) < 0
    c3 = [C3(1) C3(2)];
    [C_3,alpha_new3] = min(abs(c3-alpha1(3)));
    Alpha1(3) = c3(alpha_new3);
elseif alpha1(3) > C3(3) && alpha1(3) < C3(4) && u_d(3) > 0 || alpha1(3) > C3(3) && alpha1(3) < C3(4) && u_d(3) < 0 
    c3 = [C3(3) C3(4)];
    [C_3,alpha_new3] = min(abs(c3-alpha1(3)));
    Alpha1(3) = c3(alpha_new3);
else 
    Alpha1(3) = alpha1(3);
end
if alpha(3) > C3(1)+0.1  && alpha(3) < C3(2)-0.1 || alpha(3) > C3(3)+0.1 && alpha(3) < C3(4)-0.1
    u_d(3) = 0;
else 
    u_d(3) = u_d(3);
end

% Thruster 4 OK
%C4 = [-52.8 -34.2 52.8 34.2]; 
if alpha1(4) > C4(1)  && alpha1(4) < C4(2) && u_d(4) > 0 || alpha1(4) > C4(1)  && alpha1(4) < C4(2) && u_d(4) < 0
    c4 = [C4(1) C4(2)];
    [C_4,alpha_new4] = min(abs(c4-alpha1(4)));
    Alpha1(4) = c4(alpha_new4);
elseif alpha1(4) < C4(3) && alpha1(4) > C4(4) && u_d(4) > 0 || alpha1(4) < C4(3) && alpha1(4) > C4(4) && u_d(4) < 0 
    c4 = [C4(3) C4(4)];
    [C_4,alpha_new4] = min(abs(c4-alpha1(4)));
    Alpha1(4) = c4(alpha_new4);
else 
    Alpha1(4) = alpha1(4);
end
if alpha(4) > C4(1)+0.1  && alpha(4) < C4(2)-0.1 || alpha(4) < C4(3)-0.1 && alpha(4) > C4(4)+0.1
    u_d(4) = 0;
else 
    u_d(4) = u_d(4);
end

% Thruster 5
%C5 = [-98.25 -81.75 -145.8 -127.2];
if alpha1(5) < C5(1)  && alpha1(5) > C5(2) && u_d(5) > 0 || alpha1(5) < C5(1)  && alpha1(5) > C5(2) && u_d(5) < 0
    c5 = [C5(1) C5(2)];
    [C_5,alpha_new5] = min(abs(c5-alpha1(5)));
    Alpha1(5) = c5(alpha_new5);
elseif alpha1(5) < C5(3) && alpha1(5) > C5(4) && u_d(5) > 0  || alpha1(5) < C5(3) && alpha1(5) > C5(4) && u_d(5) < 0
    c5 = [C5(3) C5(4)];
    [C_5,alpha_new5] = min(abs(c5-alpha1(5)));
    Alpha1(5) = c5(alpha_new5);
else 
    Alpha1(5) = alpha1(5);
end
if alpha(5) < C5(1)-0.1  && alpha(5) > C5(2)+0.1 || alpha(5) < C5(3)-0.1 && alpha(5) > C5(4)+0.1
    u_d(5) = 0;
else 
    u_d(5) = u_d(5);
end

% Thruster 6
%C6 = [98.75 81.75 145.8 127.2];
if alpha1(6) > C6(1)  && alpha1(6) < C6(2) && u_d(6) > 0 || alpha1(6) > C6(1)  && alpha1(6) < C6(2) && u_d(6) < 0
    c6 = [C6(1) C6(2)];
    [C_6,alpha_new6] = min(abs(c6-alpha1(6)));
    Alpha1(6) = c6(alpha_new6);
elseif alpha1(6) > C6(3) && alpha1(6) < C6(4) && u_d(6) > 0 || alpha1(6) > C6(3) && alpha1(6) < C6(4) && u_d(6) < 0
    c6 = [C6(3) C6(4)];
    [C_6,alpha_new6] = min(abs(c6-alpha1(6)));
    Alpha1(6) = c6(alpha_new6);
else 
    Alpha1(6) = alpha1(6);
end
if alpha(6) > C6(1)+0.1  && alpha(6) < C6(2)-0.1 || alpha(6) > C6(3)+0.1 && alpha(6) < C6(4)-0.1
    u_d(6) = 0;
else 
    u_d(6) = u_d(6);
end

% Thruster 2&3 
if Alpha1(2) == C2(2)
    Alpha1(3) = alpha1(2) - (C2(2) - alpha1(2));
elseif Alpha1(2) == C2(1)
    Alpha1(3) = alpha1(2) - (C2(1) - alpha1(2));
elseif Alpha1(2) == C2(3)
    Alpha1(3) = alpha1(2) - (C2(3) - alpha1(2));
elseif Alpha1(2) == C2(4)
    Alpha1(3) = alpha1(2) - (C2(4) - alpha1(2));
    
elseif Alpha1(3) == C3(2)
    Alpha1(2) = alpha1(3) - (C3(2) - alpha1(3));
elseif Alpha1(3) == C3(1)
    Alpha1(2) = alpha1(3) - (C3(1) - alpha1(3));
elseif Alpha1(3) == C3(3)
    Alpha1(2) = alpha1(3) - (C3(3) - alpha1(3));
elseif Alpha1(3) == C3(4)
    Alpha1(2) = alpha1(3) - (C3(4) - alpha1(3));
end

% Thruster 5&6
if Alpha1(5) == C5(2)
    Alpha1(6) = alpha1(5) - (C5(2) - alpha1(5));
elseif Alpha1(5) == C5(1)
    Alpha1(6) = alpha1(5) - (C5(1) - alpha1(5));
elseif Alpha1(5) == C5(3)
    Alpha1(6) = alpha1(5) - (C5(3) - alpha1(5));
elseif Alpha1(5) == C5(4)
    Alpha1(6) = alpha1(5) - (C5(4) - alpha1(5));
    
elseif Alpha1(6) == C6(2)
    Alpha1(5) = alpha1(6) - (C6(2) - alpha1(6));
elseif Alpha1(6) == C6(1)
    Alpha1(5) = alpha1(6) - (C6(1) - alpha1(6));
elseif Alpha1(6) == C6(3)
    Alpha1(5) = alpha1(6) - (C6(3) - alpha1(6));
elseif Alpha1(6) == C6(4)
    Alpha1(5) = alpha1(6) - (C6(4) - alpha1(6));
end
% Thruster 4 & 1
if     Alpha1(4) == C4(2)
    Alpha1(1) = alpha1(4) - (C4(2) - alpha1(4));
elseif Alpha1(4) == C4(1)
    Alpha1(1) = alpha1(4) - (C4(1) - alpha1(4));
elseif Alpha1(4) == C4(3)
    Alpha1(1) = alpha1(4) - (C4(3) - alpha1(4));
elseif Alpha1(4) == C4(4)
    Alpha1(1) = alpha1(4) - (C4(4) - alpha1(4));
end

if     Alpha1(1) == C1(2)
    Alpha1(4) = alpha1(1) - (C1(2) - alpha1(1));
elseif Alpha1(1) == C1(1)
    Alpha1(4) = alpha1(1) - (C1(1) - alpha1(1));
elseif Alpha1(1) == C1(3)
    Alpha1(4) = alpha1(1) - (C1(3) - alpha1(1));
elseif Alpha1(1) == C1(4)
    Alpha1(4) = alpha1(1) - (C1(4) - alpha1(1));
end

Alpha1 = [Alpha1(1) Alpha1(2) Alpha1(3) Alpha1(4) Alpha1(5) Alpha1(6)]';    
%Desired_thrust = [u_d(1) u_d(2) u_d(3) u_d(4) u_d(5) u_d(6)]';
alpha_desired = Alpha1;


% u_d = -Desired_thrust;
%% Update outputs
sys = [alpha_desired',u_d']';

== matlab function test/Thruster control /Thrust mapped to PWM/MATLAB Function2 ==
  data: Tc_in1 input; signal input; Tc_out output; Tc_in2 input
function Tc_out = fcn(Tc_in1,signal,Tc_in2)
%#codegen

if signal >= 0
    Tc_out = Tc_in1;
else %signal < 0
    Tc_out = Tc_in2;
end

== matlab function test/Initialization of parameters/Guidance Gains/MATLAB Function ==
  data: T_x input; y output
function y = fcn(T_x)

y = 1/T_x;
